simulink model "VerificaAssegnamentoAutovalori_27042026"  (R2025b)
settings: Solver=VariableStepAuto  StartTime=0.0  StopTime=10.0  RelTol=1e-3
values from neighbouring files (symbols this model uses):
  A = double(subs(A_sym, [x; u], [x_star; u_star]))    [Esame_27042026.m]
  B = double(subs(B_sym, [x; u], [x_star; u_star]))    [Esame_27042026.m]
  C = eye(n)    [Esame_27042026.m]
  C_inseguimento_EIG = [1, 0, 0, 0, 0, 0 ... (first row only)    [Esame_27042026.m]
  D = zeros(n, m)    [Esame_27042026.m]
  K_EIG = place(A, B, eig_des)    [Esame_27042026.m]
  N = inv(C_inseguimento_EIG*(-inv(A-B*K_EIG))*B)    [Esame_27042026.m]
  x0_EIG = [0.05 ... (first row only)    [Esame_27042026.m]
  xref_EIG = [0.15 ... (first row only)    [Esame_27042026.m]
settings Model: Creator=salvo  LastModifiedBy=salvo

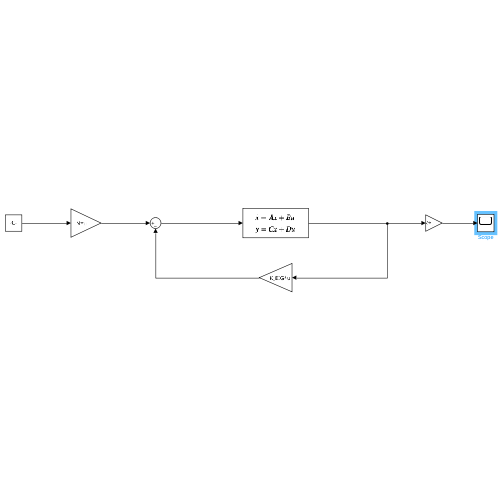
[thumbnail: Simulink's stored preview of the top-level diagram]
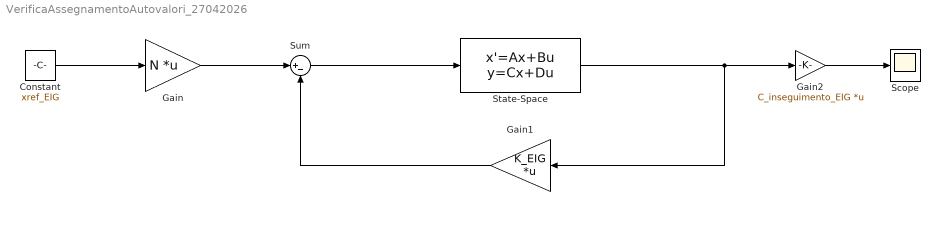
== system VerificaAssegnamentoAutovalori_27042026 ==
  Constant : Constant  Value=xref_EIG
  Gain : Gain  Gain=N  Multiplication=Matrix(K*u)
  Gain1 : Gain  Gain=K_EIG  Multiplication=Matrix(K*u)
  Gain2 : Gain  Gain=C_inseguimento_EIG  Multiplication=Matrix(K*u)
  Scope : Scope
      settings: ActiveDisplayYMinimum=-0.056967230830300891  ActiveDisplayYMaximum=0.23604631886263183
  State-Space : StateSpace  A=A  B=B  C=C  D=D  InitialCondition=x0_EIG
  Sum : Sum  Inputs=|+-
  wires:
  Sum/1 -> State-Space/1
  Gain/1 -> Sum/1
  Constant/1 -> Gain/1
  Gain1/1 -> Sum/2
  State-Space/1 -> Gain2/1, Gain1/1
  Gain2/1 -> Scope/1
